simulink model "task4"  (R2022b)
settings: Solver=FixedStepAuto  StartTime=0.0  StopTime=10.0  RelTol=1e-8
settings Model: Creator=anton  LastModifiedBy=anton
settings DataIOCC: ExternalInput=data  LoadExternalInput=on

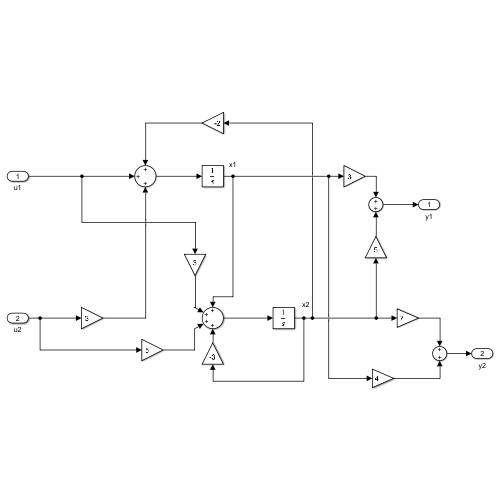
[thumbnail: Simulink's stored preview of the top-level diagram]
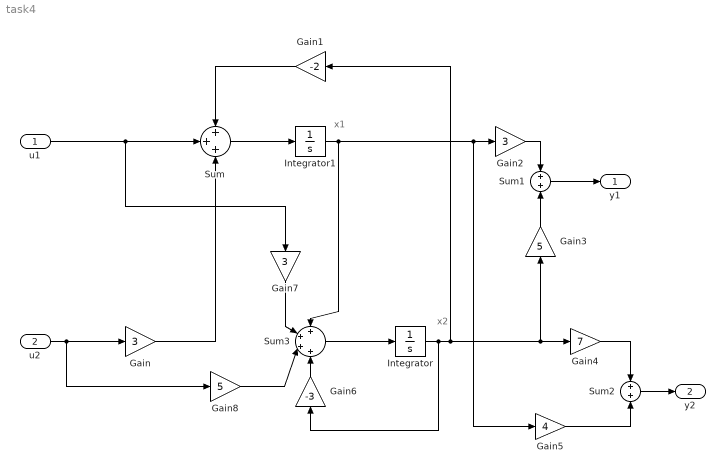
== system task4 ==
  note: x2
  note: x1
  u1 : Inport  PortDimensions=1
  u2 : Inport  Port=2  PortDimensions=1
  Gain : Gain  Gain=3
  Gain1 : Gain  Gain=-2
  Gain2 : Gain  Gain=3
  Gain3 : Gain  Gain=5
  Gain4 : Gain  Gain=7
  Gain5 : Gain  Gain=4
  Gain6 : Gain  Gain=-3
  Gain7 : Gain  Gain=3
  Gain8 : Gain  Gain=5
  Integrator : Integrator
  Integrator1 : Integrator
  Sum : Sum  Inputs=+++
  Sum1 : Sum
  Sum2 : Sum
  Sum3 : Sum  Inputs=++++
  y1 : Outport
  y2 : Outport  Port=2
  wires:
  u2/1 -> Gain8/1, Gain/1
  Gain/1 -> Sum/3
  u1/1 -> Sum/2, Gain7/1
  Integrator/1 -> Gain6/1, Gain3/1, Gain4/1, Gain1/1
  Gain1/1 -> Sum/1
  Sum/1 -> Integrator1/1
  Sum1/1 -> y1/1
  Integrator1/1 -> Sum3/1, Gain5/1, Gain2/1
  Gain2/1 -> Sum1/1
  Gain3/1 -> Sum1/2
  Sum2/1 -> y2/1
  Gain4/1 -> Sum2/1
  Gain5/1 -> Sum2/2
  Sum3/1 -> Integrator/1
  Gain6/1 -> Sum3/4
  Gain7/1 -> Sum3/2
  Gain8/1 -> Sum3/3
